simulink model "untitled"  (R2020a)
settings: Solver=ode15s  StartTime=0.0  StopTime=50  RelTol=1e-3
libraries: simulink x4, shared6dof x1
settings Model: Creator=Azriel19  LastModifiedBy=Azriel19
settings DataIOCC: SaveState=on

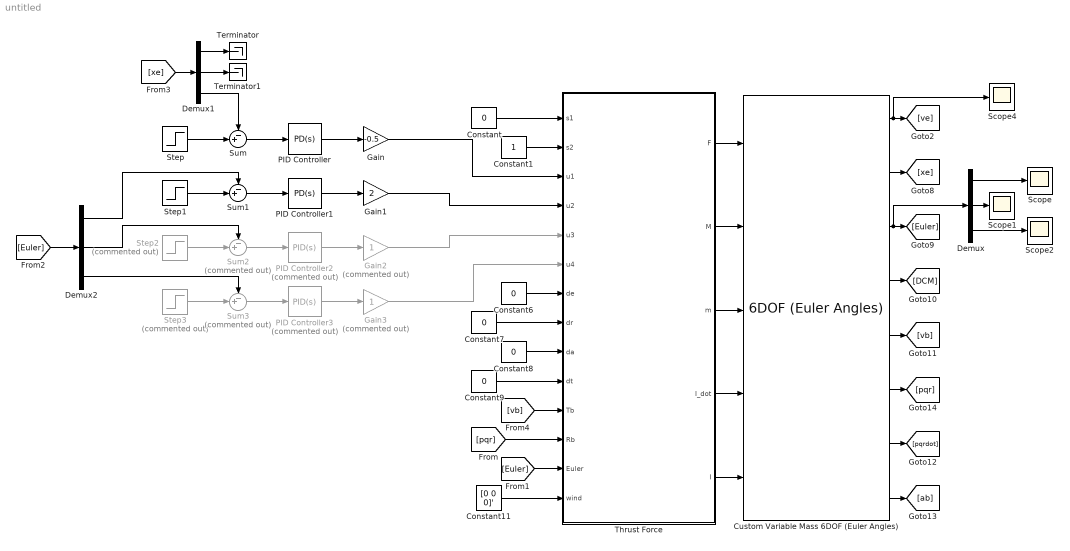
== system untitled ==
  Constant{,6..9} (5 alike) : Constant  Value=0
  Constant1 : Constant
  Constant11 : Constant  Value=[0 0 0]'
  Custom Variable Mass 6DOF (Euler Angles) : shared6dof/6DOF (Euler Angles)  units=Metric (MKS)  mtype=Custom Variable  rep=Euler Angles  xme_0=[0 0 0]  Vm_0=[0 0 0]  eul_0=[0 0 0]  pm_0=[0 0 0]  mass_0=1.0  mass_e=0.5  mass_f=2.0  inertia=eye(3)  inertia_e=eye(3)  inertia_f=2*eye(3)  k_quat=1.0  vre_flag=off  abi_flag=off  aMode=0  xme_statename=''  Vm_statename=''  eul_statename=''  quat_statename=''  pm_statename=''  mass_statename=''
      settings: SourceProductBaseCode=AE,PW,MT,VE,VP
  Demux : Demux  Outputs=3
  Demux1 : Demux  Outputs=3
  Demux2 : Demux  Outputs=3
  Gain : Gain  Gain=-0.5
  Gain1 : Gain  Gain=2
  Gain2 : Gain  Commented=on
  Gain3 : Gain  Commented=on
  PID Controller : simulink/Continuous/PID Controller  Controller=PD  Form=Parallel  TimeDomain=Continuous-time  UseExternalTs=off  SampleTime=-1  IntegratorMethod=Forward Euler  FilterMethod=Forward Euler  ControllerParametersSource=internal  P=0.1  I=1  D=10  UseFilter=on  N=100  TunerSelectOption=Transfer Function Based (PID Tuner App)  InitialConditionSource=internal  InitialConditionForIntegrator=0  InitialConditionForFilter=0  DifferentiatorICPrevScaledInput=0  ExternalReset=none  TrackingMode=off  Kt=1  LimitOutput=off  UpperSaturationLimit=inf  LowerSaturationLimit=-inf  LinearizeAsGain=on  AntiWindupMode=none  Kb=1  POutMin=[]  POutMax=[]  IOutMin=[]  IOutMax=[]  DOutMin=[]  DOutMax=[]  NOutMin=[]  NOutMax=[]  SumOutMin=[]  SumOutMax=[]  SaturationOutMin=[]  SaturationOutMax=[]  PParamMin=[]  PParamMax=[]  IParamMin=[]  IParamMax=[]  DParamMin=[]  DParamMax=[]  NParamMin=[]  NParamMax=[]  KbParamMin=[]  KbParamMax=[]  KtParamMin=[]  KtParamMax=[]  KbOutMin=[]  KbOutMax=[]  KtOutMin=[]  KtOutMax=[]  IntegratorOutMin=[]  IntegratorOutMax=[]  FilterOutMin=[]  FilterOutMax=[]  SumI1OutMin=[]  SumI1OutMax=[]  SumI2OutMin=[]  SumI2OutMax=[]  SumI3OutMin=[]  SumI3OutMax=[]  SumI4OutMin=[]  SumI4OutMax=[]  SumDOutMin=[]  SumDOutMax=[]  DifferentiatorOutMin=[]  DifferentiatorOutMax=[]  FilterDiffOutCoefMin=[]  FilterDiffOutCoefMax=[]  ReciprocalOutMin=[]  ReciprocalOutMax=[]  SumDenOutMin=[]  SumDenOutMax=[]  SumNumOutMin=[]  SumNumOutMax=[]  DivideOutMin=[]  DivideOutMax=[]  UdiffTsProdOutMin=[]  UdiffTsProdOutMax=[]  NTsProdOutMin=[]  NTsProdOutMax=[]  UintegralTsProdOutMin=[]  UintegralTsProdOutMax=[]  UngainTsProdOutMin=[]  UngainTsProdOutMax=[]  IntegratorContinuousStateAttributes=''  IntegratorStateMustResolveToSignalObject=off  IntegratorRTWStateStorageClass=Auto  FilterContinuousStateAttributes=''  FilterStateMustResolveToSignalObject=off  FilterRTWStateStorageClass=Auto  ParallelPVariant=InternalParameters  IdealPVariant=Disabled  IVariant=Disabled  DVariant=InternalParameters  IntegratorVariant=Disabled  SatVariant=Disabled  AWVariant=Disabled  PCopyVariant=Disabled  TRVariant=Disabled  FdbkBlocksVariant=Forward  IdealPFdbkVariant=Disabled  SatFdbkVariant=Disabled  DerivativeFilterVariant=ContFilter  NVariant=InternalParameters  NCopyVariant=Disabled  FilterICVariant=InternalICsFilter  IntegratorICVariant=Disabled  ExternalResetVariant=Disabled  TRSumVariant=Passthrough  SumFdbkVariant=Disabled  SumVariant=Sum_PD  TsampFilterVariant=InternalTs  TsampNgainVariant=Passthrough  TsampIntegralVariant=Disabled_SignalSpec
  PID Controller1 : simulink/Continuous/PID Controller  Controller=PD  Form=Parallel  TimeDomain=Continuous-time  UseExternalTs=off  SampleTime=-1  IntegratorMethod=Forward Euler  FilterMethod=Forward Euler  ControllerParametersSource=internal  P=1  I=1  D=0.001  UseFilter=on  N=100  TunerSelectOption=Transfer Function Based (PID Tuner App)  InitialConditionSource=internal  InitialConditionForIntegrator=0  InitialConditionForFilter=0  DifferentiatorICPrevScaledInput=0  ExternalReset=none  TrackingMode=off  Kt=1  LimitOutput=off  UpperSaturationLimit=inf  LowerSaturationLimit=-inf  LinearizeAsGain=on  AntiWindupMode=none  Kb=1  POutMin=[]  POutMax=[]  IOutMin=[]  IOutMax=[]  DOutMin=[]  DOutMax=[]  NOutMin=[]  NOutMax=[]  SumOutMin=[]  SumOutMax=[]  SaturationOutMin=[]  SaturationOutMax=[]  PParamMin=[]  PParamMax=[]  IParamMin=[]  IParamMax=[]  DParamMin=[]  DParamMax=[]  NParamMin=[]  NParamMax=[]  KbParamMin=[]  KbParamMax=[]  KtParamMin=[]  KtParamMax=[]  KbOutMin=[]  KbOutMax=[]  KtOutMin=[]  KtOutMax=[]  IntegratorOutMin=[]  IntegratorOutMax=[]  FilterOutMin=[]  FilterOutMax=[]  SumI1OutMin=[]  SumI1OutMax=[]  SumI2OutMin=[]  SumI2OutMax=[]  SumI3OutMin=[]  SumI3OutMax=[]  SumI4OutMin=[]  SumI4OutMax=[]  SumDOutMin=[]  SumDOutMax=[]  DifferentiatorOutMin=[]  DifferentiatorOutMax=[]  FilterDiffOutCoefMin=[]  FilterDiffOutCoefMax=[]  ReciprocalOutMin=[]  ReciprocalOutMax=[]  SumDenOutMin=[]  SumDenOutMax=[]  SumNumOutMin=[]  SumNumOutMax=[]  DivideOutMin=[]  DivideOutMax=[]  UdiffTsProdOutMin=[]  UdiffTsProdOutMax=[]  NTsProdOutMin=[]  NTsProdOutMax=[]  UintegralTsProdOutMin=[]  UintegralTsProdOutMax=[]  UngainTsProdOutMin=[]  UngainTsProdOutMax=[]  IntegratorContinuousStateAttributes=''  IntegratorStateMustResolveToSignalObject=off  IntegratorRTWStateStorageClass=Auto  FilterContinuousStateAttributes=''  FilterStateMustResolveToSignalObject=off  FilterRTWStateStorageClass=Auto  ParallelPVariant=InternalParameters  IdealPVariant=Disabled  IVariant=Disabled  DVariant=InternalParameters  IntegratorVariant=Disabled  SatVariant=Disabled  AWVariant=Disabled  PCopyVariant=Disabled  TRVariant=Disabled  FdbkBlocksVariant=Forward  IdealPFdbkVariant=Disabled  SatFdbkVariant=Disabled  DerivativeFilterVariant=ContFilter  NVariant=InternalParameters  NCopyVariant=Disabled  FilterICVariant=InternalICsFilter  IntegratorICVariant=Disabled  ExternalResetVariant=Disabled  TRSumVariant=Passthrough  SumFdbkVariant=Disabled  SumVariant=Sum_PD  TsampFilterVariant=InternalTs  TsampNgainVariant=Passthrough  TsampIntegralVariant=Disabled_SignalSpec
  PID Controller2 : simulink/Continuous/PID Controller  Commented=on  Controller=PID  Form=Parallel  TimeDomain=Continuous-time  UseExternalTs=off  SampleTime=-1  IntegratorMethod=Forward Euler  FilterMethod=Forward Euler  ControllerParametersSource=internal  P=1  I=1  D=0  UseFilter=on  N=100  TunerSelectOption=Transfer Function Based (PID Tuner App)  InitialConditionSource=internal  InitialConditionForIntegrator=0  InitialConditionForFilter=0  DifferentiatorICPrevScaledInput=0  ExternalReset=none  TrackingMode=off  Kt=1  LimitOutput=off  UpperSaturationLimit=inf  LowerSaturationLimit=-inf  LinearizeAsGain=on  AntiWindupMode=none  Kb=1  POutMin=[]  POutMax=[]  IOutMin=[]  IOutMax=[]  DOutMin=[]  DOutMax=[]  NOutMin=[]  NOutMax=[]  SumOutMin=[]  SumOutMax=[]  SaturationOutMin=[]  SaturationOutMax=[]  PParamMin=[]  PParamMax=[]  IParamMin=[]  IParamMax=[]  DParamMin=[]  DParamMax=[]  NParamMin=[]  NParamMax=[]  KbParamMin=[]  KbParamMax=[]  KtParamMin=[]  KtParamMax=[]  KbOutMin=[]  KbOutMax=[]  KtOutMin=[]  KtOutMax=[]  IntegratorOutMin=[]  IntegratorOutMax=[]  FilterOutMin=[]  FilterOutMax=[]  SumI1OutMin=[]  SumI1OutMax=[]  SumI2OutMin=[]  SumI2OutMax=[]  SumI3OutMin=[]  SumI3OutMax=[]  SumI4OutMin=[]  SumI4OutMax=[]  SumDOutMin=[]  SumDOutMax=[]  DifferentiatorOutMin=[]  DifferentiatorOutMax=[]  FilterDiffOutCoefMin=[]  FilterDiffOutCoefMax=[]  ReciprocalOutMin=[]  ReciprocalOutMax=[]  SumDenOutMin=[]  SumDenOutMax=[]  SumNumOutMin=[]  SumNumOutMax=[]  DivideOutMin=[]  DivideOutMax=[]  UdiffTsProdOutMin=[]  UdiffTsProdOutMax=[]  NTsProdOutMin=[]  NTsProdOutMax=[]  UintegralTsProdOutMin=[]  UintegralTsProdOutMax=[]  UngainTsProdOutMin=[]  UngainTsProdOutMax=[]  IntegratorContinuousStateAttributes=''  IntegratorStateMustResolveToSignalObject=off  IntegratorRTWStateStorageClass=Auto  FilterContinuousStateAttributes=''  FilterStateMustResolveToSignalObject=off  FilterRTWStateStorageClass=Auto  ParallelPVariant=InternalParameters  IdealPVariant=Disabled  IVariant=InternalParameters  DVariant=InternalParameters  IntegratorVariant=Continuous  SatVariant=Disabled  AWVariant=Passthrough  PCopyVariant=Disabled  TRVariant=Disabled  FdbkBlocksVariant=Forward  IdealPFdbkVariant=Disabled  SatFdbkVariant=Disabled  DerivativeFilterVariant=ContFilter  NVariant=InternalParameters  NCopyVariant=Disabled  FilterICVariant=InternalICsFilter  IntegratorICVariant=InternalICs  ExternalResetVariant=Disabled  TRSumVariant=Passthrough  SumFdbkVariant=Disabled  SumVariant=Sum_PID  TsampFilterVariant=InternalTs  TsampNgainVariant=Passthrough  TsampIntegralVariant=Passthrough
  PID Controller3 : simulink/Continuous/PID Controller  Commented=on  Controller=PID  Form=Parallel  TimeDomain=Continuous-time  UseExternalTs=off  SampleTime=-1  IntegratorMethod=Forward Euler  FilterMethod=Forward Euler  ControllerParametersSource=internal  P=1  I=1  D=0  UseFilter=on  N=100  TunerSelectOption=Transfer Function Based (PID Tuner App)  InitialConditionSource=internal  InitialConditionForIntegrator=0  InitialConditionForFilter=0  DifferentiatorICPrevScaledInput=0  ExternalReset=none  TrackingMode=off  Kt=1  LimitOutput=off  UpperSaturationLimit=inf  LowerSaturationLimit=-inf  LinearizeAsGain=on  AntiWindupMode=none  Kb=1  POutMin=[]  POutMax=[]  IOutMin=[]  IOutMax=[]  DOutMin=[]  DOutMax=[]  NOutMin=[]  NOutMax=[]  SumOutMin=[]  SumOutMax=[]  SaturationOutMin=[]  SaturationOutMax=[]  PParamMin=[]  PParamMax=[]  IParamMin=[]  IParamMax=[]  DParamMin=[]  DParamMax=[]  NParamMin=[]  NParamMax=[]  KbParamMin=[]  KbParamMax=[]  KtParamMin=[]  KtParamMax=[]  KbOutMin=[]  KbOutMax=[]  KtOutMin=[]  KtOutMax=[]  IntegratorOutMin=[]  IntegratorOutMax=[]  FilterOutMin=[]  FilterOutMax=[]  SumI1OutMin=[]  SumI1OutMax=[]  SumI2OutMin=[]  SumI2OutMax=[]  SumI3OutMin=[]  SumI3OutMax=[]  SumI4OutMin=[]  SumI4OutMax=[]  SumDOutMin=[]  SumDOutMax=[]  DifferentiatorOutMin=[]  DifferentiatorOutMax=[]  FilterDiffOutCoefMin=[]  FilterDiffOutCoefMax=[]  ReciprocalOutMin=[]  ReciprocalOutMax=[]  SumDenOutMin=[]  SumDenOutMax=[]  SumNumOutMin=[]  SumNumOutMax=[]  DivideOutMin=[]  DivideOutMax=[]  UdiffTsProdOutMin=[]  UdiffTsProdOutMax=[]  NTsProdOutMin=[]  NTsProdOutMax=[]  UintegralTsProdOutMin=[]  UintegralTsProdOutMax=[]  UngainTsProdOutMin=[]  UngainTsProdOutMax=[]  IntegratorContinuousStateAttributes=''  IntegratorStateMustResolveToSignalObject=off  IntegratorRTWStateStorageClass=Auto  FilterContinuousStateAttributes=''  FilterStateMustResolveToSignalObject=off  FilterRTWStateStorageClass=Auto  ParallelPVariant=InternalParameters  IdealPVariant=Disabled  IVariant=InternalParameters  DVariant=InternalParameters  IntegratorVariant=Continuous  SatVariant=Disabled  AWVariant=Passthrough  PCopyVariant=Disabled  TRVariant=Disabled  FdbkBlocksVariant=Forward  IdealPFdbkVariant=Disabled  SatFdbkVariant=Disabled  DerivativeFilterVariant=ContFilter  NVariant=InternalParameters  NCopyVariant=Disabled  FilterICVariant=InternalICsFilter  IntegratorICVariant=InternalICs  ExternalResetVariant=Disabled  TRSumVariant=Passthrough  SumFdbkVariant=Disabled  SumVariant=Sum_PID  TsampFilterVariant=InternalTs  TsampNgainVariant=Passthrough  TsampIntegralVariant=Passthrough
  Scope{,1..2,4} (4 alike) : Scope
  Step : Step  Time=0  After=20  SampleTime=0
  Step1 : Step  After=25  SampleTime=0
  Step2 : Step  Commented=on  SampleTime=0
  Step3 : Step  Commented=on  SampleTime=0
  Sum : Sum  Inputs=-+|
  Sum1 : Sum  Inputs=-+|
  Sum2 : Sum  Commented=on  Inputs=-+|
  Sum3 : Sum  Commented=on  Inputs=-+|
  Terminator : Terminator
  Terminator1 : Terminator
  Thrust Force : MATLAB Function  TreatAsAtomicUnit=on
  wires:
  [vb] -> Thrust Force/11(Tb)
  [Euler] -> Thrust Force/13(Euler)
  Constant11/1 -> Thrust Force/14(wind)
  Custom Variable Mass 6DOF (Euler Angles)/2 -> [xe]
  Custom Variable Mass 6DOF (Euler Angles)/6 -> [pqr]
  Custom Variable Mass 6DOF (Euler Angles)/7 -> [pqrdot]
  Custom Variable Mass 6DOF (Euler Angles)/8 -> [ab]
  Constant1/1 -> Thrust Force/2(s2)
  Custom Variable Mass 6DOF (Euler Angles)/4 -> [DCM]
  Thrust Force/4(I_dot) -> Custom Variable Mass 6DOF (Euler Angles)/4
  Thrust Force/5(I) -> Custom Variable Mass 6DOF (Euler Angles)/5
  Custom Variable Mass 6DOF (Euler Angles)/5 -> [vb]
  Thrust Force/1(F) -> Custom Variable Mass 6DOF (Euler Angles)/1
  Thrust Force/3(m) -> Custom Variable Mass 6DOF (Euler Angles)/3
  Thrust Force/2(M) -> Custom Variable Mass 6DOF (Euler Angles)/2
  Custom Variable Mass 6DOF (Euler Angles)/1 -> Scope4/1, [ve]
  Demux/1 -> Scope/1
  Demux/2 -> Scope1/1
  Demux/3 -> Scope2/1
  [pqr] -> Thrust Force/12(Rb)
  Custom Variable Mass 6DOF (Euler Angles)/3 -> Demux/1, [Euler]
  Constant9/1 -> Thrust Force/10(dt)
  Constant8/1 -> Thrust Force/9(da)
  Constant7/1 -> Thrust Force/8(dr)
  Constant6/1 -> Thrust Force/7(de)
  Constant/1 -> Thrust Force/1(s1)
  Gain/1 -> Thrust Force/3(u1)
  Gain1/1 -> Thrust Force/4(u2)
  Demux2/1 -> Sum1/1
  PID Controller3/1 -> Gain3/1
  Demux2/3 -> Sum3/1
  Sum2/1 -> PID Controller2/1
  [Euler] -> Demux2/1
  Step1/1 -> Sum1/2
  Step3/1 -> Sum3/2
  PID Controller1/1 -> Gain1/1
  Demux2/2 -> Sum2/1
  Demux1/2 -> Terminator1/1
  PID Controller/1 -> Gain/1
  Step2/1 -> Sum2/2
  Gain3/1 -> Thrust Force/6(u4)
  Gain2/1 -> Thrust Force/5(u3)
  Demux1/1 -> Terminator/1
  Step/1 -> Sum/2
  Sum1/1 -> PID Controller1/1
  Sum3/1 -> PID Controller3/1
  Demux1/3 -> Sum/1
  Sum/1 -> PID Controller/1
  [xe] -> Demux1/1
  PID Controller2/1 -> Gain2/1

== matlab function untitled/Thrust Force ==
  data: s1 input; s2 input; F output; M output; m output; I_dot output; I output; u1 input; u2 input; u3 input; u4 input; de input; dr input; da input; dt input; Tb input; Rb input; Euler input; wind input
function [F, M, m, I_dot, I] = Thrust_and_Moment(s1,s2,u1,u2,u3,u4,de,dr,da,dt,Tb,Rb,Euler,wind)

F = zeros(3,1);
M = zeros(3,1);
I = zeros(3,3);
u = Tb(1);
v = Tb(2);
w = Tb(3);
p = Rb(1);
q = Rb(2);
r = Rb(3);
roll = Euler(1);
pitch = Euler(2);
yaw = Euler(3);
w_ns = wind(1); % steady wind - North
w_es = wind(2); % steady wind - East
w_ds = wind(3); % steady wind - Down
u_wg = wind(1); % gust along body x-axis
v_wg = wind(2); % gust along body y-axis    
w_wg = wind(3); % gust along body z-axis

% compute wind data in NED
w_n = cos(pitch)*cos(yaw)*w_ns+cos(pitch)*sin(yaw)*w_es-sin(pitch)*w_ds+u_wg;
w_e = (sin(roll)*sin(pitch)*cos(yaw)-cos(roll)*sin(yaw))*w_ns+...
     (sin(roll)*sin(pitch)*sin(yaw)+cos(roll)*cos(yaw))*w_es+...
     sin(roll)*cos(pitch)*w_ds+v_wg;
w_d =(cos(roll)*sin(pitch)*cos(yaw)+sin(roll)*sin(yaw))*w_ns+...
     (cos(roll)*sin(pitch)*sin(yaw)-sin(roll)*cos(yaw))*w_es+...
     cos(roll)*cos(pitch)*w_ds+w_wg; 
 
% compute air data
ur = u-w_n; vr=v-w_e; wr=w-w_d;
Va=sqrt(ur^2+vr^2+wr^2);
if ur == 0
    ur = 0.0001;
end 
alpha = atan2(wr,ur);
if Va == 0
    Va = 0.0001;
end
B = asin(vr/Va);

% Every Parameter & Coeficient
m = 1.56; %massa
g = 9.18; %grafitasi
Ixx = 0.1147; %inertia sb x
Ixy = 0;
Ixz = 0.0015;
Iyy = 0.0576; %inertia sb y
Iyx = 0;
Iyz = 0;
Izz = 0.1712; %inertia sb z
Izx = 0.0015;
Izy = 0;
I = [Ixx Ixy Ixz; Iyx Iyy Iyz; Izx Izy Izz];
I_dot = zeros(3,3);
S = 0.2589;
b = 1.4224;
c = 0.3302;
Sprop = 0.0314;
Cprop = 1;
Kmotor = 20;
R = 1.2682;
%KTp=0;
%KOmega=0;

%Translational Coeficient
CLo = 0.09167;
CLa = 3.5026;
CLA = CLo+CLa*alpha;
CLq = 2.8932;
CLde = 0.2724;
CDo = 0.01613;
CDa = 0.2108;
CDA = CDo+CDa*alpha;
CDq = 0;
CDde=0.3045;
Cyo = 0;
Cyb = -0.07359;
Cyp = 0;
Cyr = 0;
Cyda = 0;
Cydr = -0.17;

%x-axis
Cxa = -CDA*cos(alpha)+CLA*sin(alpha);
Cxqa = -CDq*cos(alpha)+CLq*sin(alpha);
Cxdea = -CDde*cos(alpha)+CLde*sin(alpha);

%z-axis
Cza = -CDA*sin(alpha)-CLA*cos(alpha);
Czqa = -CDq*sin(alpha)-CLq*cos(alpha);
Czdea = -CDde*sin(alpha)-CLde*cos(alpha);

%Rotational Coeficient
Cmo = -0.02338;
Cma = -0.5675;
Cmq = -1.3990;
Cmde = -0.3254;
Clo = 0;
Clb = -0.02854;
Clp = -0.3209;
Clr = 0.03066;
Clda = 0.1682;
Cldr = 0.105; 
Cno = 0;
Cnb = -0.0040;
Cnp = -0.01297;
Cnr = -0.00434;
Cnda = -0.00328;
Cndr = -0.032; 

%Inertial Product
A = Ixx*Izz-Ixz^2;
%A1=(Ixz*(Ixx-Iyy+Izz))/A;
%A2=(Izz*(Izz-Iyy)+Ixz^2)/A;
A3 = Izz/A;
A4 = Ixz/A;
%A5=(Izz-Ixx)/A;
%A6=Ixz/A;
%A7=((Ixx-Iyy)*Ixx+Ixz^2)/A;
A8 = Ixx/A;

%roll 
Cpo = A3*Clo+A4*Cno;
Cpb = A3*Clb+A4*Cnb;
Cpp = A3*Clp+A4*Cnp;
Cpr = A3*Clr+A4*Cnr;
Cpda = A3*Clda+A4*Cnda;
Cpdr = A3*Cldr+A4*Cndr;

%yaw 
Cro = A4*Clo+A8*Cno;
Crb = A4*Clb+A8*Cnb;
Crp = A4*Clp+A8*Cnp;
Crr = A4*Clr+A8*Cnr;
Crda = A4*Clda+A8*Cnda;
Crdr = A4*Cldr+A8*Cndr;

%Gaya drag
Kftx = 0.0005567;
Kfty = 0.0005567;
Kftz = 0.0006354;
Kfax=0.0005567;
Kfay=0.0005567;
Kfaz=0.0006354;

%Translational
Ud = -g*sin(pitch)+s1*(R/2/m)*Va^2*S*(Cxa+Cxqa*((c*q)/(2*Va))+Cxdea*de)+s1*(R/2/m)*Sprop*Cprop*((Kmotor*dt)^2-Va^2);
%xdd = 1/m*(cos(varphi)*cos(psi)*sin(theta)+sin(psi)*sin(varphi))*u1-Kftx*u;
xdd = ((1/m)*(-Kftx)*u);

Fx = s1*m*Ud+s2*m*xdd;

vd = g*cos(pitch)*sin(roll)+s1*(R/2/m)*Va^2*S*(Cyo+Cyb*B+Cyp*(b*p/2*Va)+Cyr*(b*r/2*Va)+Cyda*da+Cydr*dr);
%ydd = 1/m*(cos(varphi)*sin(psi)*sin(theta)-cos(psi)*sin(varphi))*u1-Kfty*v;
ydd = ((1/m)*(-Kfty)*v);

Fy = s1*m*vd+s2*m*ydd;

wd = g*cos(pitch)*cos(yaw)+s1*(R/2/m)*Va^2*S*(Cza+Czqa*((c*q)/(2*Va))+Czdea*de);
%zdd = 1/m*(cos(varphi)*cos(theta))*u1-Kftz*w-g;
zdd = ((1/m)*(Kftz*w-u1));

Fz = s1*m*wd+s2*m*zdd;

F = [Fx Fy Fz]';

%Rotational
pd = (R/2*Ixx)*(Va^2*S*b)*(Cpo+Cpb*B+Cpp*(b*p/2*Va)+Cpr*(b*r/2*Va)+Cpda*da+Cpdr*dr);
%varphidd = 1/Ixx*(p*q*(Iyy-Izz)+u2-Kftz*r^2);
varphidd = (A3*(u2-Kfax*p^2)+A4*(u4-Kfaz*r^2));

Mx = s1*Ixx*pd+s2*Ixx*varphidd;

qd = (R/(2*Iyy))*(Va^2*S*c)*(Cmo+Cma*alpha+Cmq*(c*p/2*Va)+Cmde*de);
%thetadd = 1/Iyy*(r*q*(Izz-Ixx)+u3-Kftz*p^2);
thetadd = (1/Iyy)*(u3-Kfay*q^2);

My = s1*Iyy*qd+s2*Iyy*thetadd;

rd = (R/2*Izz)*(Va^2*S*b)*(Cro+Crb*B+Crp*(b*p/2*Va)+Crr*(b*r/2*Va)+Crda*da+Crdr*dr);
%psidd = 1/Izz*(p*r*(Ixx-Iyy)+u4-Kftz*q^2);
psidd = (A4*(u2-Kfax*p^2)+A8*(u4-Kfaz*r^2));

Mz = s1*Izz*rd+s2*Izz*psidd;

M = [Mx My Mz]';

%Rotation Matrix
%C = [cos(pitch)*cos(yaw) sin(roll)*sin(pitch)*cos(yaw)-cos(roll)*sin(yaw) cos(roll)*sin(pitch)*sin(yaw)+sin(roll)*sin(yaw);
    %cos(pitch)*sin(yaw) sin(roll)*sin(pitch)*sin(yaw)+cos(roll)*cos(yaw) cos(roll)*sin(pitch)*sin(yaw)-sin(roll)*cos(yaw);
    %sin(pitch) -sin(roll)*cos(pitch) -cos(roll)*cos(pitch)];

%rolldot=p+q*sin(roll)*tan(pitch)+r*cos(roll)*tan(pitch);
%pitchdot=q*cos(roll)-r*sin(roll);
%yawdot=q*sin(roll)/cos(pitch)+r*cos(roll)/cos(pitch);
%Medot = C*[u v w]';
